simulink model "PID_controller"  (R2019b)
settings: Solver=VariableStepAuto  StartTime=0.0  StopTime=10.0  RelTol=1e-3
InitFcn:
  | % generator parameters
  | A_1 = 1;
  | A_2 = 1;
  | psi_1 = 0;
  | psi_2 = 0;
  | omegaref_1 = 1;
  | omegaref_2 = 2;
  | 
  | wref_0 = [A_1*sin(psi_1) omegaref_1*A_1*cos(psi_1) A_2*sin(psi_2) omegaref_2*A_2*cos(psi_2)];
  | Sref = [0 1 0 0; -omegaref_1^2 0 0 0; 0 0 0 1; 0 0 -omegaref_2^2 0];
  | Qrefp = [1 0 0 0; 0 0 1 0];
  | Qrefv = [0 1 0 0; 0 0 0 1];
  | Qrefa = [-omegaref_1^2 0 0 0; 0 0 -omegaref_2^2 0];
  | 
  | % model parameters
  | m_1 = 1;
  | m_2 = 1;
  | l_1 = 1;
  | l_2 = 1;
  | l_c1 = 1/2;
  | l_c2 = 1/2;
  | I_1 = 1;
  | I_2 = 1;
  | g = 9.81;
  | 
  | rho_1 = m_1*l_c1^2+m_2*l_1^2+2*m_2*l_1*l_c2^2+I_1;
  | rho_2 = m_2*l_c2^2+I_2;
  | rho_3 = m_2*l_1*l_c2;
  | rho_4 = (m_1*l_c1+m_2*l_1)*g;
  | rho_5 = m_2*l_c2*g;
  | rho_6 = m_2*l_c2;
  | 
  | % friction
  | F_fric = [0.1 0; 0 0.1];
  | 
  | % proportional and derivative K
  | K_p = [100 0; 0 100];
  | K_d = [100 0; 0 100];
settings Model: Creator=Eugene  LastModifiedBy=Eugene

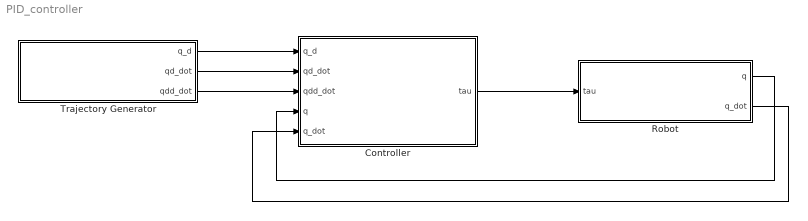
== system PID_controller ==
  Controller : Subsystem
  Robot : Subsystem
  Trajectory Generator : Subsystem
  wires:
  Controller/1(tau) -> Robot/1(tau)
  Robot/1(q) -> Controller/4(q)
  Robot/2(q_dot) -> Controller/5(q_dot)
  Trajectory Generator/1(q_d) -> Controller/1(q_d)
  Trajectory Generator/2(qd_dot) -> Controller/2(qd_dot)
  Trajectory Generator/3(qdd_dot) -> Controller/3(qdd_dot)

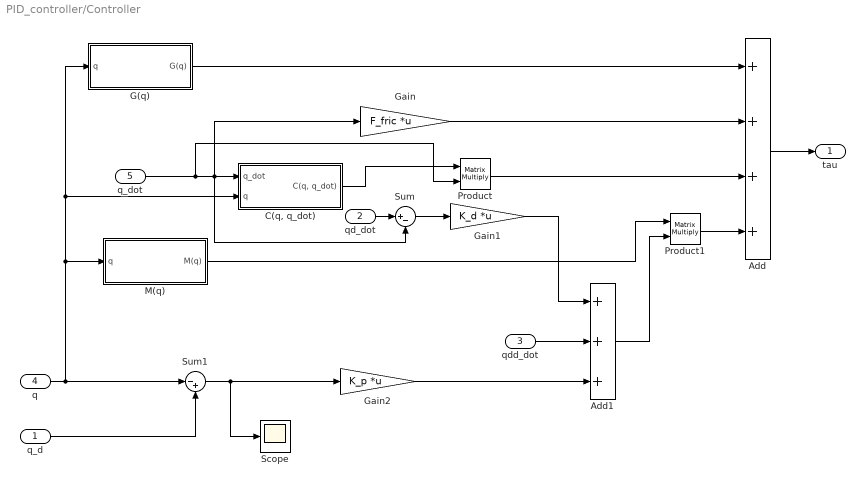
== system PID_controller/Controller ==
  q_d : Inport
  qd_dot : Inport  Port=2
  qdd_dot : Inport  Port=3
  q : Inport  Port=4
  q_dot : Inport  Port=5
  Add : Sum  Inputs=4
  Add1 : Sum  Inputs=3
  "C(q, q_dot)" : Subsystem
  G(q) : Subsystem
  Gain : Gain  Gain=F_fric  Multiplication=Matrix(K*u) (u vector)
  Gain1 : Gain  Gain=K_d  Multiplication=Matrix(K*u) (u vector)
  Gain2 : Gain  Gain=K_p  Multiplication=Matrix(K*u) (u vector)
  M(q) : Subsystem
  Product : Product  Multiplication=Matrix(*)
  Product1 : Product  Multiplication=Matrix(*)
  Scope : Scope
  Sum : Sum  Inputs=|+-
  Sum1 : Sum  Inputs=|-+
  tau : Outport
  wires:
  G(q)/1(G(q)) -> Add/1
  Gain/1 -> Add/2
  Add/1 -> tau/1
  Product/1 -> Add/3
  "C(q, q_dot)"/1("C(q, q_dot)") -> Product/1
  Add1/1 -> Product1/2
  qd_dot/1 -> Sum/1
  q_dot/1 -> Product/2, Sum/2, "C(q, q_dot)"/1(q_dot), Gain/1
  Sum/1 -> Gain1/1
  Gain1/1 -> Add1/1
  qdd_dot/1 -> Add1/2
  Gain2/1 -> Add1/3
  Sum1/1 -> Scope/1, Gain2/1
  q_d/1 -> Sum1/2
  q/1 -> Sum1/1, M(q)/1(q), "C(q, q_dot)"/2(q), G(q)/1(q)
  Product1/1 -> Add/4
  M(q)/1(M(q)) -> Product1/1

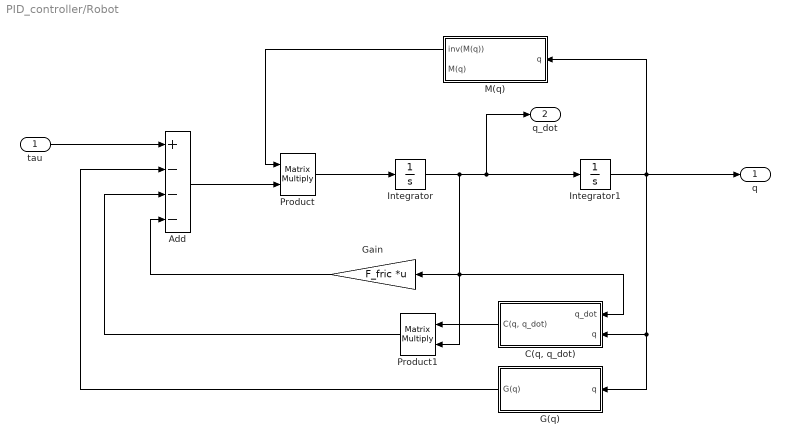
== system PID_controller/Robot ==
  tau : Inport
  Add : Sum  Inputs=+---
  "C(q, q_dot)" : Subsystem
  G(q) : Subsystem
  Gain : Gain  Gain=F_fric  Multiplication=Matrix(K*u) (u vector)
  Integrator : Integrator
  Integrator1 : Integrator
  M(q) : Subsystem
  Product : Product  Multiplication=Matrix(*)
  Product1 : Product  Multiplication=Matrix(*)
  q : Outport
  q_dot : Outport  Port=2
  wires:
  Integrator1/1 -> q/1, "C(q, q_dot)"/2(q), G(q)/1(q), M(q)/1(q)
  Integrator/1 -> "C(q, q_dot)"/1(q_dot), Product1/2, Gain/1, q_dot/1, Integrator1/1
  M(q)/1(inv(M(q))) -> Product/1
  Product1/1 -> Add/3
  tau/1 -> Add/1
  "C(q, q_dot)"/1("C(q, q_dot)") -> Product1/1
  Add/1 -> Product/2
  G(q)/1(G(q)) -> Add/2
  Product/1 -> Integrator/1
  Gain/1 -> Add/4

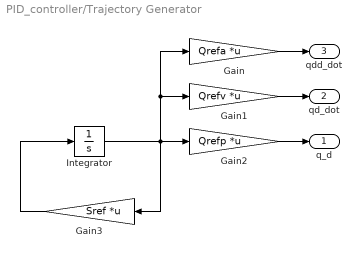
== system PID_controller/Trajectory Generator ==
  Gain : Gain  Gain=Qrefa  Multiplication=Matrix(K*u) (u vector)
  Gain1 : Gain  Gain=Qrefv  Multiplication=Matrix(K*u) (u vector)
  Gain2 : Gain  Gain=Qrefp  Multiplication=Matrix(K*u) (u vector)
  Gain3 : Gain  Gain=Sref  Multiplication=Matrix(K*u) (u vector)
  Integrator : Integrator  InitialCondition=wref_0
  q_d : Outport
  qd_dot : Outport  Port=2
  qdd_dot : Outport  Port=3
  wires:
  Gain3/1 -> Integrator/1
  Integrator/1 -> Gain3/1, Gain1/1, Gain/1, Gain2/1
  Gain2/1 -> q_d/1
  Gain1/1 -> qd_dot/1
  Gain/1 -> qdd_dot/1

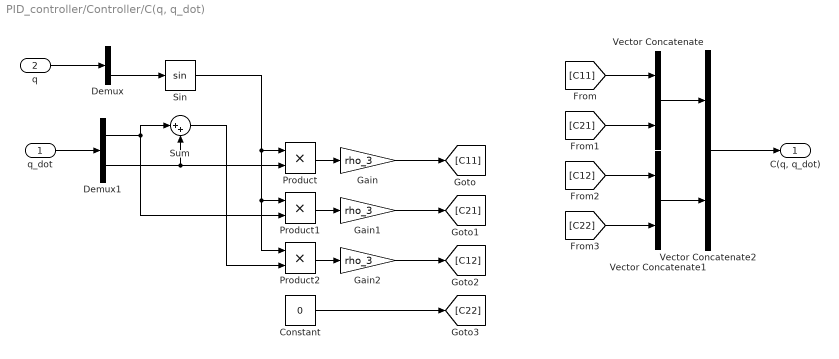
== system PID_controller/Controller/C(q, q_dot) ==
  q_dot : Inport
  q : Inport  Port=2
  Constant : Constant  Value=0
  Demux : Demux  Outputs=2
  Demux1 : Demux  Outputs=2
  Gain : Gain  Gain=rho_3
  Gain1 : Gain  Gain=rho_3
  Gain2 : Gain  Gain=rho_3
  Product : Product
  Product1 : Product
  Product2 : Product
  Sin : Trigonometry
  Sum : Sum  Inputs=|++
  Vector Concatenate : Concatenate
  Vector Concatenate1 : Concatenate
  Vector Concatenate2 : Concatenate  Mode=Multidimensional array  ConcatenateDimension=2
  "C(q, q_dot)" : Outport
  wires:
  q/1 -> Demux/1
  q_dot/1 -> Demux1/1
  Demux1/1 -> Sum/1, Product1/2
  Sin/1 -> Product/1, Product2/1, Product1/1
  Demux1/2 -> Product/2, Sum/2
  Sum/1 -> Product2/2
  Product/1 -> Gain/1
  Product1/1 -> Gain1/1
  Product2/1 -> Gain2/1
  Gain/1 -> [C11]
  Gain1/1 -> [C21]
  Gain2/1 -> [C12]
  Constant/1 -> [C22]
  [C12] -> Vector Concatenate1/1
  [C22] -> Vector Concatenate1/2
  [C21] -> Vector Concatenate/2
  [C11] -> Vector Concatenate/1
  Vector Concatenate2/1 -> "C(q, q_dot)"/1
  Vector Concatenate/1 -> Vector Concatenate2/1
  Vector Concatenate1/1 -> Vector Concatenate2/2
  Demux/2 -> Sin/1

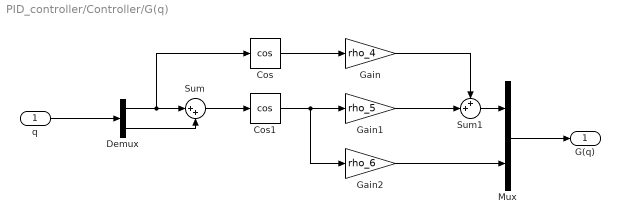
== system PID_controller/Controller/G(q) ==
  q : Inport
  Cos : Trigonometry  Operator=cos
  Cos1 : Trigonometry  Operator=cos
  Demux : Demux  Outputs=2
  Gain : Gain  Gain=rho_4
  Gain1 : Gain  Gain=rho_5
  Gain2 : Gain  Gain=rho_6
  Mux : Mux  Inputs=2
  Sum : Sum  Inputs=|++
  Sum1 : Sum  Inputs=++|
  G(q) : Outport
  wires:
  q/1 -> Demux/1
  Demux/1 -> Cos/1, Sum/1
  Demux/2 -> Sum/2
  Sum/1 -> Cos1/1
  Cos/1 -> Gain/1
  Cos1/1 -> Gain2/1, Gain1/1
  Gain/1 -> Sum1/1
  Gain1/1 -> Sum1/2
  Sum1/1 -> Mux/1
  Gain2/1 -> Mux/2
  Mux/1 -> G(q)/1

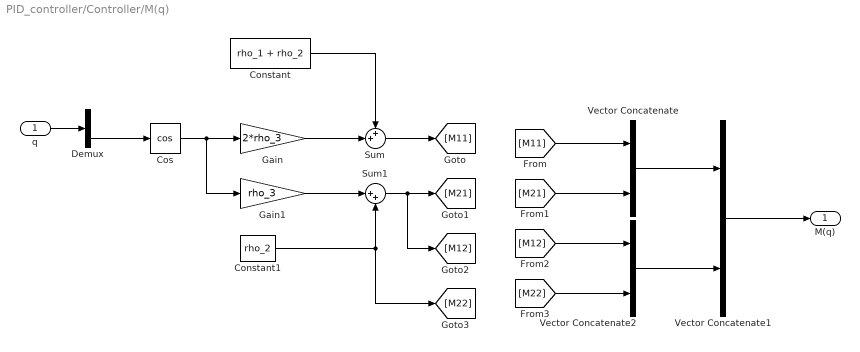
== system PID_controller/Controller/M(q) ==
  q : Inport
  Constant : Constant  Value=rho_1 + rho_2
  Constant1 : Constant  Value=rho_2
  Cos : Trigonometry  Operator=cos
  Demux : Demux  Outputs=2
  Gain : Gain  Gain=2*rho_3
  Gain1 : Gain  Gain=rho_3
  Sum : Sum  Inputs=++|
  Sum1 : Sum  Inputs=|++
  Vector Concatenate : Concatenate
  Vector Concatenate1 : Concatenate  Mode=Multidimensional array  ConcatenateDimension=2
  Vector Concatenate2 : Concatenate
  M(q) : Outport
  wires:
  Demux/2 -> Cos/1
  Gain/1 -> Sum/2
  Vector Concatenate1/1 -> M(q)/1
  [M21] -> Vector Concatenate/2
  [M12] -> Vector Concatenate2/1
  [M22] -> Vector Concatenate2/2
  Gain1/1 -> Sum1/1
  [M11] -> Vector Concatenate/1
  q/1 -> Demux/1
  Sum/1 -> [M11]
  Vector Concatenate/1 -> Vector Concatenate1/1
  Constant1/1 -> [M22], Sum1/2
  Constant/1 -> Sum/1
  Sum1/1 -> [M12], [M21]
  Cos/1 -> Gain1/1, Gain/1
  Vector Concatenate2/1 -> Vector Concatenate1/2

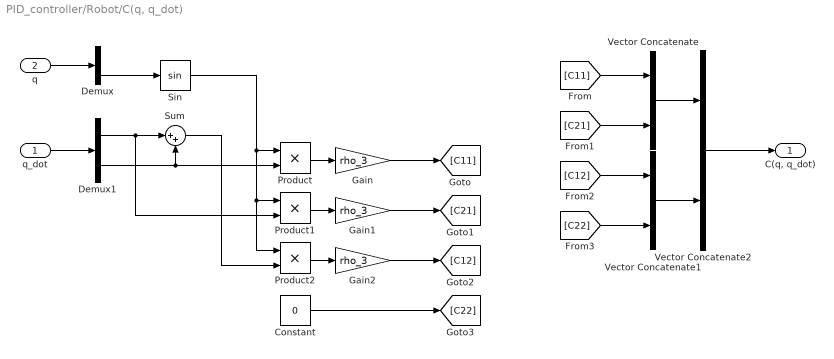
== system PID_controller/Robot/C(q, q_dot) ==
  q_dot : Inport
  q : Inport  Port=2
  Constant : Constant  Value=0
  Demux : Demux  Outputs=2
  Demux1 : Demux  Outputs=2
  Gain : Gain  Gain=rho_3
  Gain1 : Gain  Gain=rho_3
  Gain2 : Gain  Gain=rho_3
  Product : Product
  Product1 : Product
  Product2 : Product
  Sin : Trigonometry
  Sum : Sum  Inputs=|++
  Vector Concatenate : Concatenate
  Vector Concatenate1 : Concatenate
  Vector Concatenate2 : Concatenate  Mode=Multidimensional array  ConcatenateDimension=2
  "C(q, q_dot)" : Outport
  wires:
  q/1 -> Demux/1
  q_dot/1 -> Demux1/1
  Demux1/1 -> Sum/1, Product1/2
  Sin/1 -> Product/1, Product2/1, Product1/1
  Demux1/2 -> Product/2, Sum/2
  Sum/1 -> Product2/2
  Product/1 -> Gain/1
  Product1/1 -> Gain1/1
  Product2/1 -> Gain2/1
  Gain/1 -> [C11]
  Gain1/1 -> [C21]
  Gain2/1 -> [C12]
  Constant/1 -> [C22]
  [C12] -> Vector Concatenate1/1
  [C22] -> Vector Concatenate1/2
  [C21] -> Vector Concatenate/2
  [C11] -> Vector Concatenate/1
  Vector Concatenate2/1 -> "C(q, q_dot)"/1
  Vector Concatenate/1 -> Vector Concatenate2/1
  Vector Concatenate1/1 -> Vector Concatenate2/2
  Demux/2 -> Sin/1

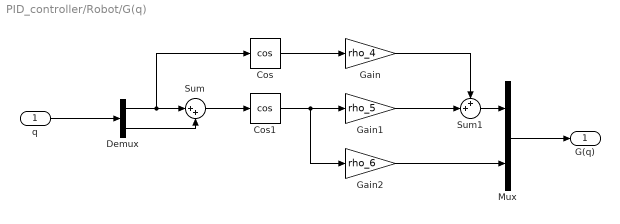
== system PID_controller/Robot/G(q) ==
  q : Inport
  Cos : Trigonometry  Operator=cos
  Cos1 : Trigonometry  Operator=cos
  Demux : Demux  Outputs=2
  Gain : Gain  Gain=rho_4
  Gain1 : Gain  Gain=rho_5
  Gain2 : Gain  Gain=rho_6
  Mux : Mux  Inputs=2
  Sum : Sum  Inputs=|++
  Sum1 : Sum  Inputs=++|
  G(q) : Outport
  wires:
  q/1 -> Demux/1
  Demux/1 -> Cos/1, Sum/1
  Demux/2 -> Sum/2
  Sum/1 -> Cos1/1
  Cos/1 -> Gain/1
  Cos1/1 -> Gain2/1, Gain1/1
  Gain/1 -> Sum1/1
  Gain1/1 -> Sum1/2
  Sum1/1 -> Mux/1
  Gain2/1 -> Mux/2
  Mux/1 -> G(q)/1

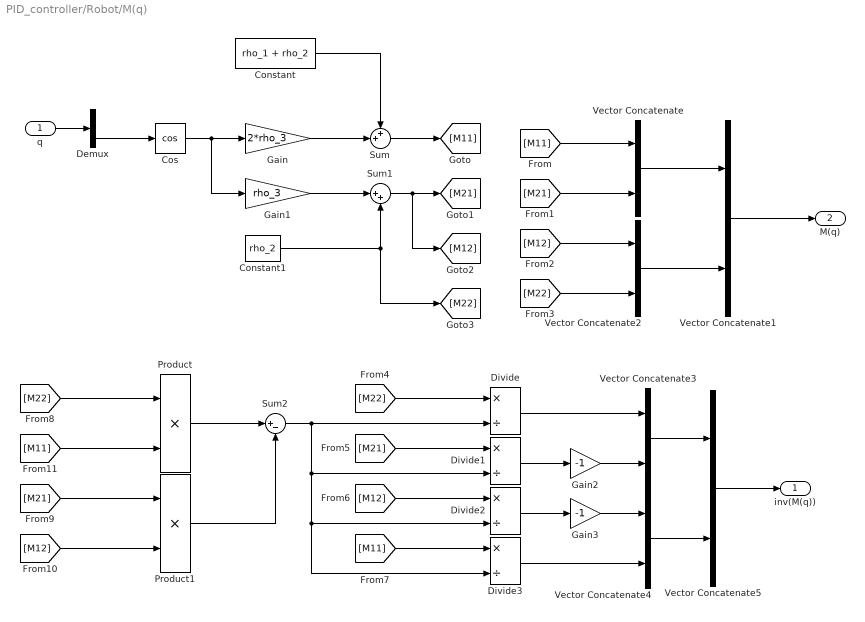
== system PID_controller/Robot/M(q) ==
  q : Inport
  Constant : Constant  Value=rho_1 + rho_2
  Constant1 : Constant  Value=rho_2
  Cos : Trigonometry  Operator=cos
  Demux : Demux  Outputs=2
  Divide{,1..3} (4 alike) : Product  Inputs=*/
  Gain : Gain  Gain=2*rho_3
  Gain1 : Gain  Gain=rho_3
  Gain2 : Gain  Gain=-1
  Gain3 : Gain  Gain=-1
  Product : Product
  Product1 : Product
  Sum : Sum  Inputs=++|
  Sum1 : Sum  Inputs=|++
  Sum2 : Sum  Inputs=|+-
  Vector Concatenate : Concatenate
  Vector Concatenate1 : Concatenate  Mode=Multidimensional array  ConcatenateDimension=2
  Vector Concatenate2 : Concatenate
  Vector Concatenate3 : Concatenate  Mode=Multidimensional array  ConcatenateDimension=2
  Vector Concatenate4 : Concatenate  Mode=Multidimensional array  ConcatenateDimension=2
  Vector Concatenate5 : Concatenate  Mode=Multidimensional array
  inv(M(q)) : Outport
  M(q) : Outport  Port=2
  wires:
  q/1 -> Demux/1
  Cos/1 -> Gain1/1, Gain/1
  Gain/1 -> Sum/2
  Constant/1 -> Sum/1
  Sum1/1 -> [M12], [M21]
  Sum/1 -> [M11]
  Gain1/1 -> Sum1/1
  Constant1/1 -> [M22], Sum1/2
  [M21] -> Product1/1
  [M11] -> Product/2
  [M12] -> Product1/2
  [M22] -> Product/1
  Product/1 -> Sum2/1
  Product1/1 -> Sum2/2
  [M21] -> Divide1/1
  [M22] -> Divide/1
  [M11] -> Divide3/1
  [M12] -> Divide2/1
  Sum2/1 -> Divide1/2, Divide2/2, Divide3/2, Divide/2
  Divide1/1 -> Gain2/1
  Divide2/1 -> Gain3/1
  Divide/1 -> Vector Concatenate3/1
  Gain2/1 -> Vector Concatenate3/2
  Divide3/1 -> Vector Concatenate4/2
  Gain3/1 -> Vector Concatenate4/1
  Vector Concatenate3/1 -> Vector Concatenate5/1
  Vector Concatenate4/1 -> Vector Concatenate5/2
  Vector Concatenate5/1 -> inv(M(q))/1
  [M11] -> Vector Concatenate/1
  [M22] -> Vector Concatenate2/2
  [M12] -> Vector Concatenate2/1
  [M21] -> Vector Concatenate/2
  Vector Concatenate/1 -> Vector Concatenate1/1
  Vector Concatenate2/1 -> Vector Concatenate1/2
  Vector Concatenate1/1 -> M(q)/1
  Demux/2 -> Cos/1
